simulink model "Proyecto_Motor_Control_Velocidad"  (R2017b)
settings: Solver=VariableStepAuto  StartTime=0.0  StopTime=5  MaxStep=1e-4  RelTol=1e-3
values from neighbouring files (symbols this model uses):
  Ts = 2e-3    (= 0.002)    [Ploteo_Datos.m]
undefined symbols (not defined in the file or in its folder): Jm, Ke, Kt, La, Ra, Vcc
libraries: powerlib x16, simulink x3, dspstat3 x1, powerlib_meascontrol x1
settings Model: Creator=ezema  LastModifiedBy=ezema

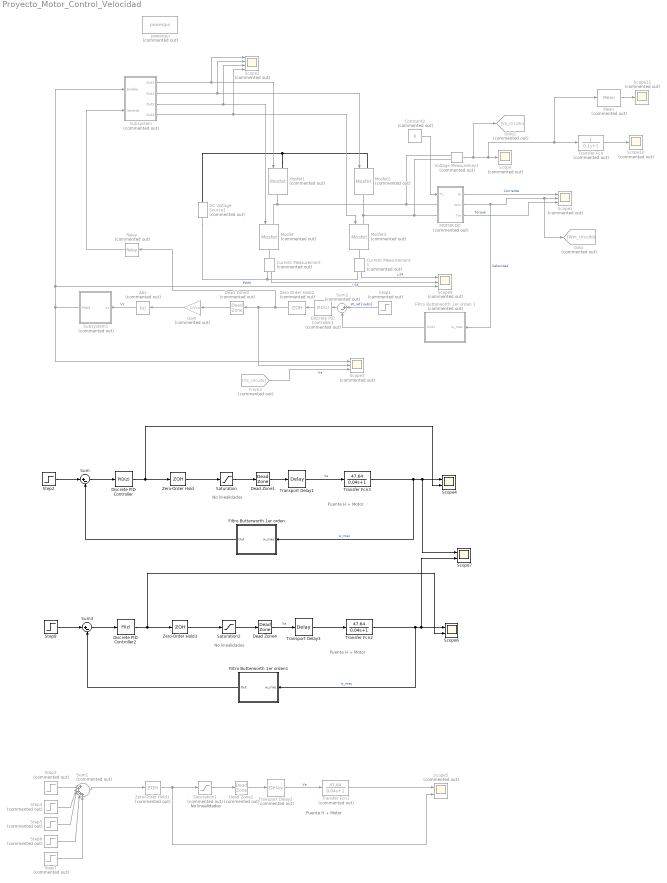
== system Proyecto_Motor_Control_Velocidad ==
  note: Puente H + Motor
  note: No linealidades
  note: Puente H + Motor
  note: No linealidades
  note: No linealidades
  note: Puente H + Motor
  Abs : Abs  Commented=on
  Constant2 : Constant  Commented=on  Value=0
  Current Measurement : powerlib/Measurements/Current Measurement  Commented=on  PhasorSimulation=off  OutputType=Complex  PSBequivalent=0
  Current Measurement1 : powerlib/Measurements/Current Measurement  Commented=on  PhasorSimulation=off  OutputType=Complex  PSBequivalent=0
  DC Voltage Source1 : powerlib/Electrical Sources/DC Voltage Source  Commented=on  Amplitude=Vcc  Measurements=None
  Dead Zone1 : DeadZone  LowerValue=-8.5  UpperValue=8.5  SaturateOnIntegerOverflow=on
  Dead Zone2 : DeadZone  Commented=on  LowerValue=-8.5  UpperValue=8.5  SaturateOnIntegerOverflow=on
  Dead Zone3 : DeadZone  Commented=on  LowerValue=-8.5  UpperValue=8.5  SaturateOnIntegerOverflow=on
  Dead Zone4 : DeadZone  LowerValue=-8.5  UpperValue=8.5  SaturateOnIntegerOverflow=on
  Discrete PID Controller : simulink/Continuous/PID Controller  Controller=PID  TimeDomain=Discrete-time  SampleTime=-1  IntegratorMethod=Forward Euler  FilterMethod=Forward Euler  Form=Ideal  UseFilter=off  ControllerParametersSource=internal  P=0.00123  I=200  D=0  N=100  InitialConditionSource=internal  InitialConditionForIntegrator=0  InitialConditionForFilter=0  ExternalReset=none  LimitOutput=off  UpperSaturationLimit=inf  LowerSaturationLimit=-inf  LinearizeAsGain=off  AntiWindupMode=none  Kb=1  TrackingMode=off  Kt=1  PParamMin=[]  PParamMax=[]  IParamMin=[]  IParamMax=[]  DParamMin=[]  DParamMax=[]  NParamMin=[]  NParamMax=[]  KbParamMin=[]  KbParamMax=[]  KtParamMin=[]  KtParamMax=[]  POutMin=[]  POutMax=[]  IOutMin=[]  IOutMax=[]  DOutMin=[]  DOutMax=[]  NOutMin=[]  NOutMax=[]  KbOutMin=[]  KbOutMax=[]  KtOutMin=[]  KtOutMax=[]  IntegratorOutMin=[]  IntegratorOutMax=[]  FilterOutMin=[]  FilterOutMax=[]  SumOutMin=[]  SumOutMax=[]  SumI1OutMin=[]  SumI1OutMax=[]  SumI2OutMin=[]  SumI2OutMax=[]  SumI3OutMin=[]  SumI3OutMax=[]  SumDOutMin=[]  SumDOutMax=[]  SaturationOutMin=[]  SaturationOutMax=[]  IntegratorContinuousStateAttributes=''  IntegratorStateMustResolveToSignalObject=off  IntegratorRTWStateStorageClass=Auto  FilterContinuousStateAttributes=''  FilterStateMustResolveToSignalObject=off  FilterRTWStateStorageClass=Auto  DifferentiatorICPrevScaledInput=0  DifferentiatorOutMin=[]  DifferentiatorOutMax=[]  InitialConditionSetting=State (most efficient)  FilterDiffOutCoefMin=[]  FilterDiffOutCoefMax=[]  SumDenOutMin=[]  SumDenOutMax=[]  SumNumOutMin=[]  SumNumOutMax=[]  ReciprocalOutMin=[]  ReciprocalOutMax=[]  DivideOutMin=[]  DivideOutMax=[]  TunerSelectOption=Frequency Response Based
  Discrete PID Controller1 : simulink/Continuous/PID Controller  Commented=on  Controller=PID  TimeDomain=Discrete-time  SampleTime=-1  IntegratorMethod=Forward Euler  FilterMethod=Forward Euler  Form=Parallel  UseFilter=on  ControllerParametersSource=internal  P=0.05  I=0  D=0  N=100  InitialConditionSource=internal  InitialConditionForIntegrator=0  InitialConditionForFilter=0  ExternalReset=none  LimitOutput=off  UpperSaturationLimit=inf  LowerSaturationLimit=-inf  LinearizeAsGain=off  AntiWindupMode=none  Kb=1  TrackingMode=off  Kt=1  PParamMin=[]  PParamMax=[]  IParamMin=[]  IParamMax=[]  DParamMin=[]  DParamMax=[]  NParamMin=[]  NParamMax=[]  KbParamMin=[]  KbParamMax=[]  KtParamMin=[]  KtParamMax=[]  POutMin=[]  POutMax=[]  IOutMin=[]  IOutMax=[]  DOutMin=[]  DOutMax=[]  NOutMin=[]  NOutMax=[]  KbOutMin=[]  KbOutMax=[]  KtOutMin=[]  KtOutMax=[]  IntegratorOutMin=[]  IntegratorOutMax=[]  FilterOutMin=[]  FilterOutMax=[]  SumOutMin=[]  SumOutMax=[]  SumI1OutMin=[]  SumI1OutMax=[]  SumI2OutMin=[]  SumI2OutMax=[]  SumI3OutMin=[]  SumI3OutMax=[]  SumDOutMin=[]  SumDOutMax=[]  SaturationOutMin=[]  SaturationOutMax=[]  IntegratorContinuousStateAttributes=''  IntegratorStateMustResolveToSignalObject=off  IntegratorRTWStateStorageClass=Auto  FilterContinuousStateAttributes=''  FilterStateMustResolveToSignalObject=off  FilterRTWStateStorageClass=Auto  DifferentiatorICPrevScaledInput=0  DifferentiatorOutMin=[]  DifferentiatorOutMax=[]  InitialConditionSetting=State (most efficient)  FilterDiffOutCoefMin=[]  FilterDiffOutCoefMax=[]  SumDenOutMin=[]  SumDenOutMax=[]  SumNumOutMin=[]  SumNumOutMax=[]  ReciprocalOutMin=[]  ReciprocalOutMax=[]  DivideOutMin=[]  DivideOutMax=[]  TunerSelectOption=Transfer Function Based (PID Tuner App)
  Discrete PID Controller2 : simulink/Continuous/PID Controller  Controller=PI  TimeDomain=Discrete-time  SampleTime=Ts  IntegratorMethod=Forward Euler  FilterMethod=Forward Euler  Form=Ideal  UseFilter=off  ControllerParametersSource=internal  P=0.00123  I=450/2  D=4.99965142913872e-06  N=100  InitialConditionSource=internal  InitialConditionForIntegrator=0  InitialConditionForFilter=0  ExternalReset=none  LimitOutput=off  UpperSaturationLimit=inf  LowerSaturationLimit=-inf  LinearizeAsGain=off  AntiWindupMode=none  Kb=1  TrackingMode=off  Kt=1  PParamMin=[]  PParamMax=[]  IParamMin=[]  IParamMax=[]  DParamMin=[]  DParamMax=[]  NParamMin=[]  NParamMax=[]  KbParamMin=[]  KbParamMax=[]  KtParamMin=[]  KtParamMax=[]  POutMin=[]  POutMax=[]  IOutMin=[]  IOutMax=[]  DOutMin=[]  DOutMax=[]  NOutMin=[]  NOutMax=[]  KbOutMin=[]  KbOutMax=[]  KtOutMin=[]  KtOutMax=[]  IntegratorOutMin=[]  IntegratorOutMax=[]  FilterOutMin=[]  FilterOutMax=[]  SumOutMin=[]  SumOutMax=[]  SumI1OutMin=[]  SumI1OutMax=[]  SumI2OutMin=[]  SumI2OutMax=[]  SumI3OutMin=[]  SumI3OutMax=[]  SumDOutMin=[]  SumDOutMax=[]  SaturationOutMin=[]  SaturationOutMax=[]  IntegratorContinuousStateAttributes=''  IntegratorStateMustResolveToSignalObject=off  IntegratorRTWStateStorageClass=Auto  FilterContinuousStateAttributes=''  FilterStateMustResolveToSignalObject=off  FilterRTWStateStorageClass=Auto  DifferentiatorICPrevScaledInput=0  DifferentiatorOutMin=[]  DifferentiatorOutMax=[]  InitialConditionSetting=State (most efficient)  FilterDiffOutCoefMin=[]  FilterDiffOutCoefMax=[]  SumDenOutMin=[]  SumDenOutMax=[]  SumNumOutMin=[]  SumNumOutMax=[]  ReciprocalOutMin=[]  ReciprocalOutMax=[]  DivideOutMin=[]  DivideOutMax=[]  TunerSelectOption=Transfer Function Based (PID Tuner App)
  Filtro Butterworth 1er orden : Subsystem
  Filtro Butterworth 1er orden 1 : Subsystem  Commented=on
  Filtro Butterworth 1er orden1 : Subsystem
  From2 : From  Commented=on  GotoTag=Va_circuito
  Gain : Gain  Commented=on  Gain=1/Vcc
  Goto : Goto  Commented=on  GotoTag=Wm_circuito
  Goto1 : Goto  Commented=on  GotoTag=Va_circuito
  "MOTOR DC " : Subsystem  Commented=on
  Mean : dspstat3/Mean  Commented=on  run=off  reset_popup=None  InputProcessing=Columns as channels (frame based)  directionMode=Each column  dimension=1  roiEnable=off  roiType=Rectangles  roiPortion=Entire ROI  roiOutput=Individual statistics for each ROI  roiFlag=off  outputDataTypeStr=Inherit: Same as accumulator  outputLastDataTypeStr=Inherit: Same as accumulator  outputMin=[]  outputMax=[]  roundingMode=Floor  overflowMode=off
  Mosfet{,1..3} (4 alike) : powerlib/Power Electronics/Mosfet  Commented=on  Ron=0  Lon=0  Rd=0  Vfd=0  IC=0  Rs=inf  Cs=inf  Measurements=off
  Relay : Relay  Commented=on  OnSwitchValue=0.001  OffSwitchValue=-0.1
  Saturation : Saturate  UpperLimit=17  LowerLimit=-17
  Saturation1 : Saturate  Commented=on  UpperLimit=17  LowerLimit=-17
  Saturation2 : Saturate  UpperLimit=17  LowerLimit=-17
  Scope : Scope  Commented=on
  Scope1 : Scope  Commented=on  NumInputPorts=3
  Scope10 : Scope  Commented=on
  Scope11 : Scope  Commented=on
  Scope2 : Scope  Commented=on  NumInputPorts=4
  Scope3 : Scope  Commented=on  NumInputPorts=3
  Scope4 : Scope  NumInputPorts=2
  Scope5 : Scope  Commented=on  NumInputPorts=2
  Scope6 : Scope  NumInputPorts=2
  Scope7 : Scope  NumInputPorts=2
  Scope9 : Scope  Commented=on  NumInputPorts=3
  Step1 : Step  Commented=on  Before=200  After=300  SampleTime=0
  Step2 : Step  Time=2  Before=200  After=300  SampleTime=0
  Step3 : Step  Commented=on  Time=2  Before=9.3114  After=10.6416  SampleTime=0
  Step4 : Step  Commented=on  Time=4  After=1.3302  SampleTime=0
  Step5 : Step  Commented=on  Time=6  After=1.3302  SampleTime=0
  Step6 : Step  Commented=on  Time=8  After=1.3302  SampleTime=0
  Step7 : Step  Commented=on  Time=10  After=1.3302  SampleTime=0
  Step8 : Step  Time=2  Before=200  After=300  SampleTime=0
  Subsystem : Subsystem  Commented=on
  Subsystem1 : Subsystem  Commented=on
  Sum : Sum  Inputs=|+-
  Sum1 : Sum  Commented=on  Inputs=|+++++
  Sum2 : Sum  Commented=on  Inputs=|+-
  Sum3 : Sum  Inputs=|+-
  Transfer Fcn : TransferFcn  Commented=on  Denominator=[0.1 1]
  Transfer Fcn1 : TransferFcn  Commented=on  Numerator=[47.64]  Denominator=[0.04 1]
  Transfer Fcn2 : TransferFcn  Numerator=[47.64]  Denominator=[0.04 1]
  Transfer Fcn3 : TransferFcn  Numerator=[47.64]  Denominator=[0.04 1]
  Transport Delay1 : TransportDelay  DelayTime=1*Ts
  Transport Delay2 : TransportDelay  Commented=on  DelayTime=1*Ts
  Transport Delay3 : TransportDelay  DelayTime=1*Ts
  Voltage Measurement : powerlib/Measurements/Voltage Measurement  Commented=on  PhasorSimulation=off  OutputType=Complex  PSBequivalent=0
  Zero-Order Hold : ZeroOrderHold  SampleTime=Ts
  Zero-Order Hold1 : ZeroOrderHold  Commented=on  SampleTime=Ts
  Zero-Order Hold2 : ZeroOrderHold  Commented=on  SampleTime=Ts
  Zero-Order Hold3 : ZeroOrderHold  SampleTime=Ts
  powergui : powerlib/powergui  Priority=1  Commented=on  SimulationMode=Continuous  SampleTime=50e-6  frequency=60  Iterations=50  frequencyindice=0  Pbase=100e6  ErrMax=1e-4  UnitsV=kV  UnitsW=MW  buscounter=0  FunctionMessages=off  echomessages=off  EnableUseOfTLC=off  CurrentSourceSwitches=off  DisableSnubberDevices=off  DisableRonSwitches=off  DisableVfSwitches=off  DisplayEquations=off  SolverType=Tustin/Backward Euler (TBE)  Interpol=off  ExternalGateDelay=off  methode=off  Ts=100  x0status=blocks  SPID=on  SwTol=0  HookPort=off  RestoreLinks=warning  ResistiveCurrentMeasurement=off  Frange=[0:2:500]  Ylog=off  Xlog=on  ShowGrid=off  save=off  variable=ZData  structure=0  ZoomFFT=off  StartTime=0.0  cycles=1  DisplayStyle=1  fundamental=60  FreqAxis=off  MaxFrequency=1000  frequencyindicesteady=1  RmsSteady=1  display=off
  wires:
  Subsystem/4("Out4 ") -> Mosfet3/1, Scope2/4
  Constant2/1 -> "MOTOR DC "/1(TL)
  Subsystem/3("Out3 ") -> Mosfet/1, Scope2/3
  Subsystem/1(Out1) -> Scope2/1, Mosfet1/1
  Subsystem/2(Out2) -> Scope2/2, Mosfet2/1
  "MOTOR DC "/1(Ia) -> Scope1/1  "Corriente"
  "MOTOR DC "/2(Wm) -> Filtro Butterworth 1er orden 1/1(w_mec), Goto/1, Scope1/2  "Velocidad"
  "MOTOR DC "/3(Tm) -> Scope1/3  "Torque"
  Step2/1 -> Sum/1
  Transfer Fcn3/1 -> Scope7/1, Scope4/1, Filtro Butterworth 1er orden/1(w_mec)  "w_mec"
  Step1/1 -> Sum2/1  "W_ref [rad/s]"
  Subsystem1/1("PWM ") -> Scope3/1, Scope9/3, Subsystem/1(Enable)  "PWM"
  From2/1 -> Scope3/3  "Va"
  Current Measurement1/1 -> Scope9/1  "i_S4"
  Current Measurement/1 -> Scope9/2  "i_S3"
  Relay/1 -> Subsystem/2(Sentido)
  Voltage Measurement/1 -> Goto1/1, Mean/1, Transfer Fcn/1, Scope/1
  Gain/1 -> Abs/1
  Transfer Fcn/1 -> Scope10/1
  Mean/1 -> Scope11/1
  Filtro Butterworth 1er orden 1/1(Out1) -> Sum2/2
  Zero-Order Hold2/1 -> Scope3/2, Dead Zone3/1, Relay/1
  Abs/1 -> Subsystem1/1(Vc)  "Vc"
  Dead Zone3/1 -> Gain/1
  Saturation/1 -> Dead Zone1/1
  Dead Zone1/1 -> Transport Delay1/1
  Sum/1 -> Discrete PID Controller/1
  Discrete PID Controller/1 -> Zero-Order Hold/1, Scope4/2
  Transport Delay1/1 -> Transfer Fcn3/1  "Va"
  Zero-Order Hold/1 -> Saturation/1
  Transport Delay2/1 -> Transfer Fcn1/1  "Va"
  Zero-Order Hold1/1 -> Scope5/2, Saturation1/1
  Dead Zone2/1 -> Transport Delay2/1
  Saturation1/1 -> Dead Zone2/1
  Transfer Fcn1/1 -> Scope5/1
  Step3/1 -> Sum1/1
  Sum1/1 -> Zero-Order Hold1/1
  Step4/1 -> Sum1/2
  Step5/1 -> Sum1/3
  Step6/1 -> Sum1/4
  Step7/1 -> Sum1/5
  Filtro Butterworth 1er orden/1(Out) -> Sum/2
  Discrete PID Controller1/1 -> Zero-Order Hold2/1
  Sum2/1 -> Discrete PID Controller1/1
  Saturation2/1 -> Dead Zone4/1
  Zero-Order Hold3/1 -> Saturation2/1
  Step8/1 -> Sum3/1
  Discrete PID Controller2/1 -> Zero-Order Hold3/1, Scope6/2
  Sum3/1 -> Discrete PID Controller2/1
  Filtro Butterworth 1er orden1/1(Out) -> Sum3/2
  Transfer Fcn2/1 -> Scope7/2, Scope6/1, Filtro Butterworth 1er orden1/1(w_mec)  "w_mec"
  Transport Delay3/1 -> Transfer Fcn2/1
  Dead Zone4/1 -> Transport Delay3/1  "Va"
  connections:
  Mosfet1/LConn1 -- Mosfet2/LConn1 -- DC Voltage Source1/RConn1
  Mosfet1/RConn1 -- Mosfet/LConn1 -- Voltage Measurement/LConn1 -- "MOTOR DC "/LConn1
  Mosfet2/RConn1 -- Mosfet3/LConn1 -- Voltage Measurement/LConn2 -- "MOTOR DC "/LConn2
  Current Measurement/LConn1 -- Mosfet/RConn1
  Current Measurement1/LConn1 -- Mosfet3/RConn1
  Current Measurement1/RConn1 -- DC Voltage Source1/LConn1 -- Current Measurement/RConn1

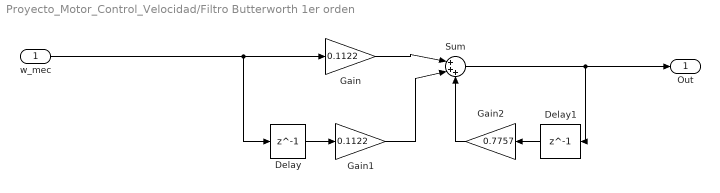
== system Proyecto_Motor_Control_Velocidad/Filtro Butterworth 1er orden ==
  w_mec : Inport
  Delay : Delay  DelayLength=1  SampleTime=Ts
  Delay1 : Delay  DelayLength=1  SampleTime=Ts
  Gain : Gain  Gain=0.1122
  Gain1 : Gain  Gain=0.1122
  Gain2 : Gain  Gain=0.7757
  Sum : Sum  Inputs=|+++
  Out : Outport
  wires:
  Gain2/1 -> Sum/3
  Delay1/1 -> Gain2/1
  Gain/1 -> Sum/1
  Delay/1 -> Gain1/1
  w_mec/1 -> Gain/1, Delay/1
  Sum/1 -> Out/1, Delay1/1
  Gain1/1 -> Sum/2

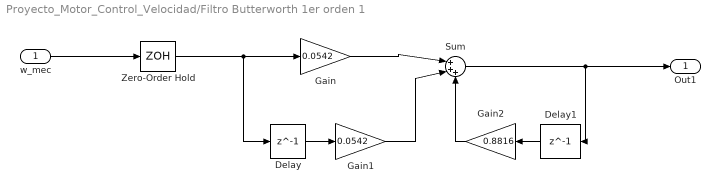
== system Proyecto_Motor_Control_Velocidad/Filtro Butterworth 1er orden 1 ==
  w_mec : Inport
  Delay : Delay  DelayLength=1  SampleTime=Ts
  Delay1 : Delay  DelayLength=1  SampleTime=Ts
  Gain : Gain  Gain=0.0542
  Gain1 : Gain  Gain=0.0542
  Gain2 : Gain  Gain=0.8816
  Sum : Sum  Inputs=|+++
  Zero-Order Hold : ZeroOrderHold  SampleTime=Ts
  Out1 : Outport
  wires:
  Gain2/1 -> Sum/3
  Delay1/1 -> Gain2/1
  Gain/1 -> Sum/1
  Delay/1 -> Gain1/1
  Zero-Order Hold/1 -> Gain/1, Delay/1
  Sum/1 -> Out1/1, Delay1/1
  Gain1/1 -> Sum/2
  w_mec/1 -> Zero-Order Hold/1

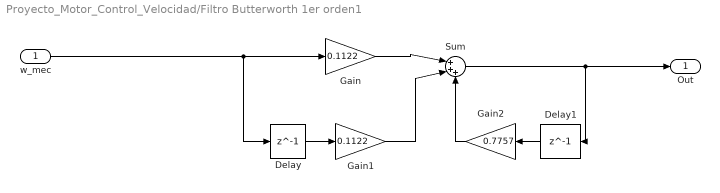
== system Proyecto_Motor_Control_Velocidad/Filtro Butterworth 1er orden1 ==
  w_mec : Inport
  Delay : Delay  DelayLength=1  SampleTime=Ts
  Delay1 : Delay  DelayLength=1  SampleTime=Ts
  Gain : Gain  Gain=0.1122
  Gain1 : Gain  Gain=0.1122
  Gain2 : Gain  Gain=0.7757
  Sum : Sum  Inputs=|+++
  Out : Outport
  wires:
  Gain2/1 -> Sum/3
  Delay1/1 -> Gain2/1
  Gain/1 -> Sum/1
  Delay/1 -> Gain1/1
  w_mec/1 -> Gain/1, Delay/1
  Sum/1 -> Out/1, Delay1/1
  Gain1/1 -> Sum/2

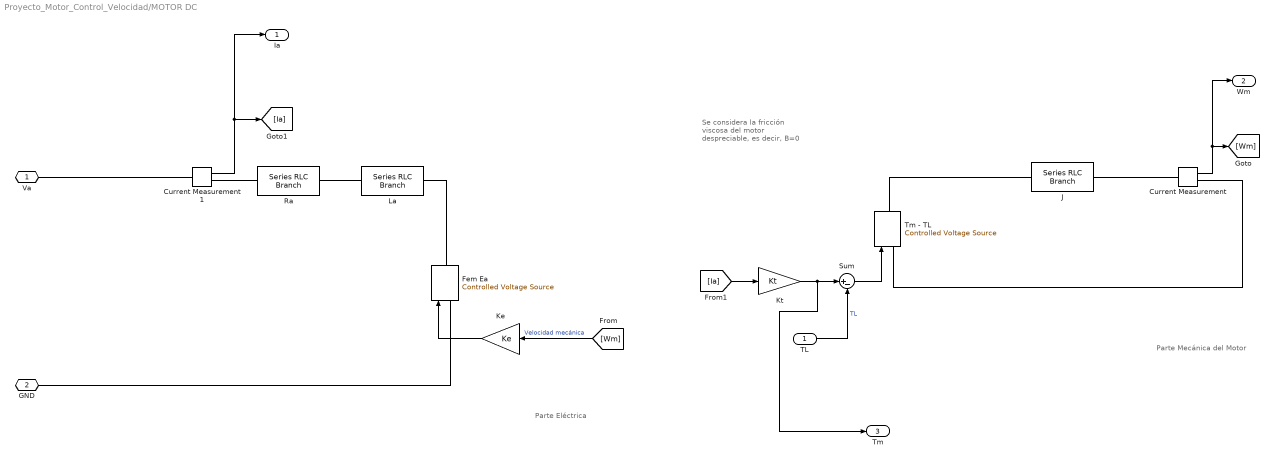
== system Proyecto_Motor_Control_Velocidad/MOTOR DC  ==
  note: Se considera la fricción viscosa del motor despreciable, es decir, B=0
  note: Parte Eléctrica
  note: Parte Mecánica del Motor
  TL : Inport
  " Fem Ea" : powerlib/Electrical Sources/Controlled Voltage Source  Initialize=on  Source_Type=DC  Amplitude=0  Phase=0  Frequency=0  Measurements=None
  " Tm - TL" : powerlib/Electrical Sources/Controlled Voltage Source  Initialize=on  Source_Type=DC  Amplitude=0  Phase=0  Frequency=0  Measurements=None
  Current Measurement : powerlib/Measurements/Current Measurement  PhasorSimulation=off  OutputType=Complex  PSBequivalent=0
  Current Measurement1 : powerlib/Measurements/Current Measurement  PhasorSimulation=off  OutputType=Complex  PSBequivalent=0
  J : powerlib/Elements/Series RLC Branch  LConnTagsString=__new0  RConnTagsString=__new0  BranchType=L  Resistance=1  Inductance=Jm  SetiL0=off  InitialCurrent=0  Capacitance=1e-6  Setx0=off  InitialVoltage=0  Measurements=None
  Ke : Gain  Gain=Ke
  Kt : Gain  Gain=Kt
  La : powerlib/Elements/Series RLC Branch  LConnTagsString=__new0  RConnTagsString=__new0  BranchType=L  Resistance=1  Inductance=La  SetiL0=off  InitialCurrent=0  Capacitance=1e-6  Setx0=off  InitialVoltage=0  Measurements=None
  Ra : powerlib/Elements/Series RLC Branch  LConnTagsString=__new0  RConnTagsString=__new0  BranchType=R  Resistance=Ra  Inductance=1e-3  SetiL0=off  InitialCurrent=0  Capacitance=1e-6  Setx0=off  InitialVoltage=0  Measurements=None
  Sum : Sum  Inputs=|+-
  Va : PMIOPort  Port=1  Side=Left
  GND : PMIOPort  Port=2  Side=Left
  Ia : Outport
  Wm : Outport  Port=2
  Tm : Outport  Port=3
  wires:
  Sum/1 -> " Tm - TL"/1
  TL/1 -> Sum/2  "TL"
  [Wm] -> Ke/1  "Velocidad mecánica"
  Current Measurement1/1 -> Ia/1, [Ia]
  Kt/1 -> Tm/1, Sum/1
  Ke/1 -> " Fem Ea"/1
  [Ia] -> Kt/1
  Current Measurement/1 -> Wm/1, [Wm]
  connections:
  Current Measurement/RConn1 -- " Tm - TL"/LConn1
  Current Measurement1/RConn1 -- Ra/LConn1
  Current Measurement/LConn1 -- J/RConn1
  Va/RConn1 -- Current Measurement1/LConn1
  " Fem Ea"/LConn1 -- GND/RConn1
  " Tm - TL"/RConn1 -- J/LConn1
  La/LConn1 -- Ra/RConn1
  La/RConn1 -- " Fem Ea"/RConn1

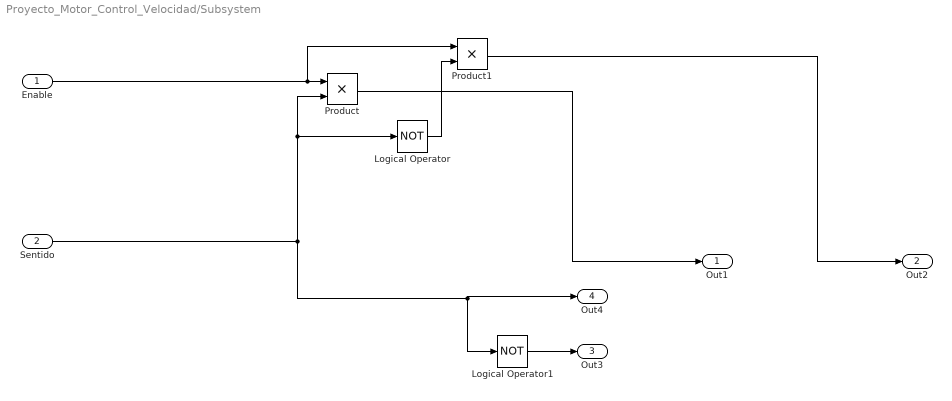
== system Proyecto_Motor_Control_Velocidad/Subsystem ==
  Enable : Inport
  Sentido : Inport  Port=2
  Logical Operator : Logic  Operator=NOT  AllPortsSameDT=off  OutDataTypeStr=boolean
  Logical Operator1 : Logic  Operator=NOT  AllPortsSameDT=off  OutDataTypeStr=boolean
  Product : Product
  Product1 : Product
  Out1 : Outport
  Out2 : Outport  Port=2
  "Out3 " : Outport  Port=3
  "Out4 " : Outport  Port=4
  wires:
  Logical Operator/1 -> Product1/2
  Enable/1 -> Product1/1, Product/1
  Product/1 -> Out1/1
  Product1/1 -> Out2/1
  Sentido/1 -> Logical Operator1/1, "Out4 "/1, Logical Operator/1, Product/2
  Logical Operator1/1 -> "Out3 "/1

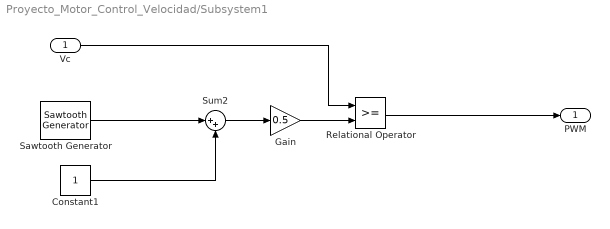
== system Proyecto_Motor_Control_Velocidad/Subsystem1 ==
  Vc : Inport
  Constant1 : Constant
  Gain : Gain  Gain=0.5
  Relational Operator : RelationalOperator  OutDataTypeStr=boolean  RndMeth=Round
  Sawtooth Generator : powerlib_meascontrol/Pulse & Signal Generators/Sawtooth Generator  Freq=20e3  Phase=0  Ts=0
      settings: SourceProductName=Simscape Power Systems
  Sum2 : Sum  Inputs=|++
  "PWM " : Outport
  wires:
  Vc/1 -> Relational Operator/1
  Relational Operator/1 -> "PWM "/1
  Constant1/1 -> Sum2/2
  Sawtooth Generator/1 -> Sum2/1
  Gain/1 -> Relational Operator/2
  Sum2/1 -> Gain/1
